simulink model "model_2151_3DOF_v3"  (Simulink 7.8)
settings: Solver=ode45  StartTime=0.0  StopTime=t_sim  FixedStep=t_step  RelTol=1e-3
values from neighbouring files (symbols this model uses):
  A_COMP = [Aq-Bq*K_lqr_int(:,1:8)-L_lqe*Cq, -Bq*K_lqr_int(:,9:10) ... (first row only)    [code_2151.m]
  Aq = [A B*Cm; zeros(2,6) Am]    [code_2151.m]
  B_COMP = [zeros(8,2), L_lqe; [1 0; 0 1], [0 -1 0; 0 0 -1]]    [code_2151.m]
  Bq = [zeros(6,2); Bm]    [code_2151.m]
  C_COMP = -K_lqr_int    [code_2151.m]
  Cq = [C zeros(3,2)]    [code_2151.m]
  D_COMP = [zeros(2,5)]    [code_2151.m]
  Dq = zeros(3,2)    [code_2151.m]
  r_psi = 170*pi/180    (= 2.96705972839)    [code_2151.m]
  r_theta = 40*pi/180    (= 0.698131700798)    [code_2151.m]
  t_noise = 0.1    [code_2151.m]
  t_psi = 10    [code_2151.m]
  t_theta = 2    [code_2151.m]
  V_sat = 4160    [code_2151.m]
libraries: commnoisgen2 x1
settings Model: Creator=lifeofsacrifice  LastModifiedBy=Dan

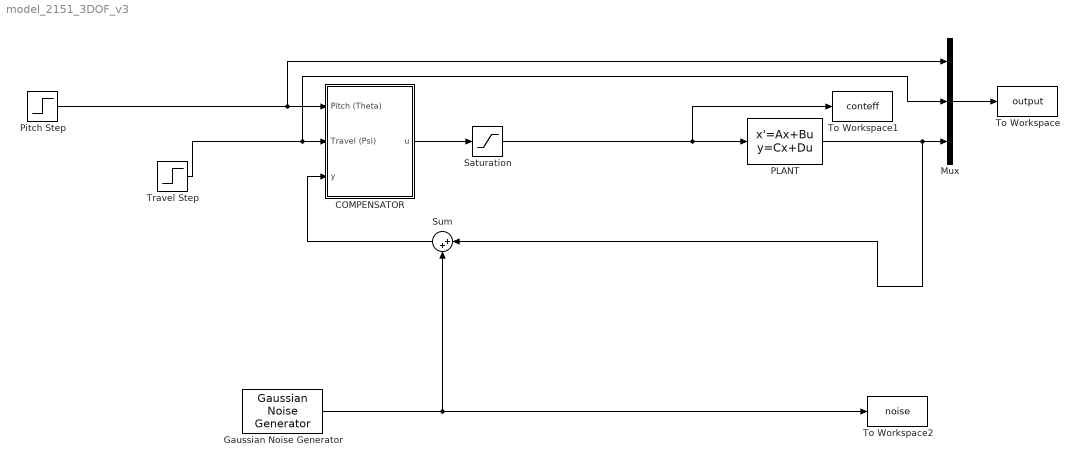
== system model_2151_3DOF_v3 ==
  COMPENSATOR : Subsystem
  Gaussian Noise Generator : commnoisgen2/Gaussian Noise Generator  m=0  d=noise_var  s=41  Ts=t_noise  frameBased=off  sampPerFrame=1  orient=off  outDataType=double
  Mux : Mux  Inputs=3
  PLANT : StateSpace  A=Aq  B=Bq  C=Cq  D=Dq
  Pitch Step : Step  Time=t_theta  After=r_theta  SampleTime=0
  Saturation : Saturate  UpperLimit=V_sat  LowerLimit=-V_sat
  Sum : Sum  Inputs=|++
  To Workspace : ToWorkspace  VariableName=output  SampleTime=-1  SaveFormat=Structure With Time
  To Workspace1 : ToWorkspace  VariableName=conteff  SampleTime=-1  SaveFormat=Structure With Time
  To Workspace2 : ToWorkspace  VariableName=noise  SampleTime=-1  SaveFormat=Structure With Time
  Travel Step : Step  Time=t_psi  After=r_psi  SampleTime=0
  wires:
  PLANT/1 -> Mux/3, Sum/1
  COMPENSATOR/1(u) -> Saturation/1
  Gaussian Noise Generator/1 -> Sum/2, To Workspace2/1
  Pitch Step/1 -> COMPENSATOR/1(Pitch (Theta)), Mux/1
  Travel Step/1 -> COMPENSATOR/2(Travel (Psi)), Mux/2
  Sum/1 -> COMPENSATOR/3(y)
  Mux/1 -> To Workspace/1
  Saturation/1 -> PLANT/1, To Workspace1/1

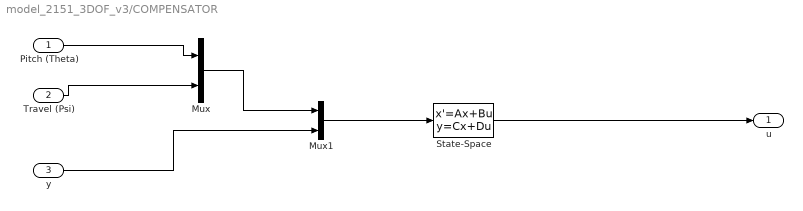
== system model_2151_3DOF_v3/COMPENSATOR ==
  Pitch (Theta) : Inport
  Travel (Psi) : Inport  Port=2
  y : Inport  Port=3
  Mux : Mux  Inputs=2
  Mux1 : Mux  Inputs=2
  State-Space : StateSpace  A=A_COMP  B=B_COMP  C=C_COMP  D=D_COMP
  u : Outport
  wires:
  Pitch (Theta)/1 -> Mux/1
  Travel (Psi)/1 -> Mux/2
  Mux/1 -> Mux1/1
  y/1 -> Mux1/2
  Mux1/1 -> State-Space/1
  State-Space/1 -> u/1
